simulink model "p6a_model"  (Simulink 8.7)
settings: Solver=FixedStepAuto  StartTime=0.0  StopTime=10.0  FixedStep=0.02  RelTol=1e-3
settings Model: Creator=eispin  LastModifiedBy=eispin
settings SolverCC: AutoInsertRateTranBlk=on
settings DataIOCC: SaveFormat=Dataset
settings DebuggingCC: UnderspecifiedInitializationDetection=Simplified  MergeDetectMultiDrivingBlocksExec=error  AllowSymbolicDim=off
settings HardwareCC: ProdBitPerPointer=64  ProdLargestAtomicFloat=Float  ProdIntDivRoundTo=Zero  ProdEndianess=LittleEndian  ProdWordSize=64  ProdHWDeviceType=Intel->x86-64 (Windows64)
settings ModelReferenceCC: PropagateSignalLabelsOutOfModel=on
settings GRTTargetCC: GeneratePreprocessorConditionals=Use local settings
settings ConfigComp: CovModelRefEnable=off

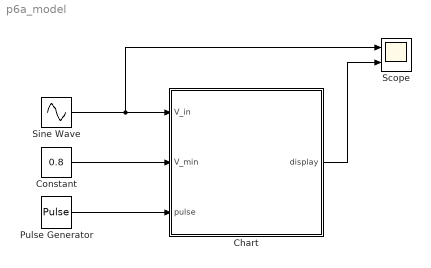
== system p6a_model ==
  Chart : Stateflow chart  TreatAsAtomicUnit=on
  Constant : Constant  Value=0.8
  Pulse Generator : DiscretePulseGenerator  PulseType=Time based  Period=1  PulseWidth=50
  Scope : Scope  NumInputPorts=2
  Sine Wave : Sin  Frequency=2.3*2*pi  SampleTime=0
  wires:
  Constant/1 -> Chart/2(V_min)
  Sine Wave/1 -> Scope/1, Chart/1(V_in)
  Chart/1(display) -> Scope/2
  Pulse Generator/1 -> Chart/3(pulse)

== stateflow chart Chart ==
  settings: enableNonTerminalStates=1
  state s
  s -> s [order 2] : [(p_sense == 1) && (V_in >= V_min)]
      | {counter = counter + 1; p_sense = 0}
  s -> s [order 1] : [(p_sense == 0) && (V_in < V_min)]
      | {p_sense = 1}
  (default) -> s : {counter = 0,	p_sense = 1,
      |   display = 0,	t_sense = 1  }
  s -> s [order 4] : [t_sense == 1 && pulse > 0.5]
      | {display=counter; counter = 0; t_sense = 0}
  s -> s [order 3] : [t_sense == 0 && pulse < 0.5]
      | {t_sense = 1}
  data: V_in input double; V_min input double; display output double; counter local double; pulse input double; t_sense local double; p_sense local double
